simulink model "kunal_project"  (R2024b)
settings: Solver=VariableStepAuto  StartTime=0.0  StopTime=5  RelTol=1e-3
undefined symbols (not defined in the file or in its folder): Ion, Lithium
libraries: spsSeriesRLCBranchLib x12, spsCurrentMeasurementLib x10, slpidlib x9, spsDiodeLib x6, spsIdealSwitchLib x6, spsPWMGeneratorDCDCLib x4, spsVoltageMeasurementLib x4, spsBatteryLib x2, spsBreakerLib x2, spsPVArrayLib x2, eeStairGenerator x2, spspowerguiLib x1
(part 2 of 2)

== matlab function kunal_project/Subsystem/MATLAB Function1 ==
  settings: updateMethod=DISCRETE
  data: Param input; Vref output; Enabled input; V input; I input
function Vref  = PandO(Param, Enabled, V, I)

% MPPT controller based on the Perturb & Observe algorithm.

% D output = Reference for DC link voltage (Vdc_ref) 
%
% Enabled input = 1 to enable the MPPT controller
% V input = PV array terminal voltage (V)
% I input = PV array current (A)
%
% Param input:
Dinit = Param(1);  %Initial value for Vdc_ref
Dmax = Param(2);   %Maximum value for Vdc_ref
Dmin = Param(3);   %Minimum value for Vdc_ref
deltaD = Param(4); %Increment value used to increase/decrease Vdc_ref
%  

persistent Vold Pold volt_old;

dataType = 'double';

if isempty(Vold)
    Vold=0;
    Pold=0;
    volt_old=Dinit;
end
P= V*I;
dV= V - Vold;
dP= P - Pold;

if dP ~= 0 & Enabled ~=0
    if dP < 0
        if dV < 0
            Vref = volt_old + deltaD;
        else
            Vref = volt_old - deltaD;
        end
    else
        if dV < 0
            Vref = volt_old - deltaD;
        else
            Vref = volt_old + deltaD;
        end    
    end
else Vref=volt_old;
end

if Vref >= Dmax | Vref<= Dmin
    Vref=volt_old;
end

volt_old=Vref;
Vold=V;
Pold=P;

== matlab function kunal_project/MATLAB Function ==
  settings: updateMethod=DISCRETE
  data: Param input; Vref output; Enabled input; V input; I input
function Vref  = PandO(Param, Enabled, V, I)

% MPPT controller based on the Perturb & Observe algorithm.

% D output = Reference for DC link voltage (Vdc_ref) 
%
% Enabled input = 1 to enable the MPPT controller
% V input = PV array terminal voltage (V)
% I input = PV array current (A)
%
% Param input:
Dinit = Param(1);  %Initial value for Vdc_ref
Dmax = Param(2);   %Maximum value for Vdc_ref
Dmin = Param(3);   %Minimum value for Vdc_ref
deltaD = Param(4); %Increment value used to increase/decrease Vdc_ref
%  

persistent Vold Pold volt_old;

dataType = 'double';

if isempty(Vold)
    Vold=0;
    Pold=0;
    volt_old=Dinit;
end
P= V*I;
dV= V - Vold;
dP= P - Pold;

if dP ~= 0 & Enabled ~=0
    if dP < 0
        if dV < 0
            Vref = volt_old + deltaD;
        else
            Vref = volt_old - deltaD;
        end
    else
        if dV < 0
            Vref = volt_old - deltaD;
        else
            Vref = volt_old + deltaD;
        end    
    end
else Vref=volt_old;
end

if Vref >= Dmax | Vref<= Dmin
    Vref=volt_old;
end

volt_old=Vref;
Vold=V;
Pold=P;
